simulink model "svlvspr1_schema_kyvadlo"  (R2018b)
settings: Solver=VariableStepAuto  StartTime=0.0  StopTime=10  RelTol=1e-3
values from neighbouring files (symbols this model uses):
  B = 1    [svlvspr1_skript_kyvadlo.m]
  g = 10    [svlvspr1_skript_kyvadlo.m]
  k1 = -2    [svlvspr1_skript_SVLVS.m]    (also in svlvspr1_skript_kyvadlo.m = 2)
  k2 = -4    [svlvspr1_skript_SVLVS.m]    (also in svlvspr1_skript_kyvadlo.m = 2.99)
  L = 10    [svlvspr1_skript_kyvadlo.m]
  m = 1    [svlvspr1_skript_kyvadlo.m]
  r = pi    (= 3.14159265359)    [svlvspr1_skript_SVLVS.m]    (also in svlvspr1_skript_kyvadlo.m = 1.0471975512)
settings Model: Creator=Evka  LastModifiedBy=Evka

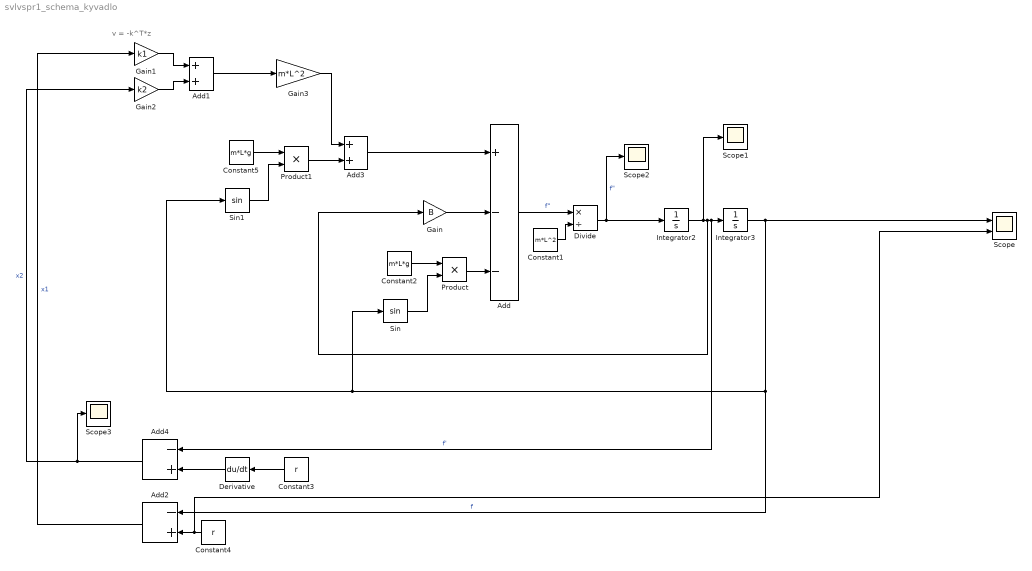
== system svlvspr1_schema_kyvadlo ==
  note: v = -k^T*z
  Add : Sum  Inputs=+--
  Add1 : Sum
  Add2 : Sum  Inputs=-+
  Add3 : Sum
  Add4 : Sum  Inputs=-+
  Constant1 : Constant  Value=m*L^2
  Constant2 : Constant  Value=m*L*g
  Constant3 : Constant  Value=r
  Constant4 : Constant  Value=r
  Constant5 : Constant  Value=m*L*g
  Derivative : Derivative
  Divide : Product  Inputs=*/
  Gain : Gain  Gain=B
  Gain1 : Gain  Gain=k1
  Gain2 : Gain  Gain=k2
  Gain3 : Gain  Gain=m*L^2
  Integrator2 : Integrator
  Integrator3 : Integrator
  Product : Product
  Product1 : Product
  Scope : Scope  NumInputPorts=2
  Scope1 : Scope
  Scope2 : Scope
  Scope3 : Scope
  Sin : Trigonometry
  Sin1 : Trigonometry
  wires:
  Add3/1 -> Add/1
  Divide/1 -> Scope2/1, Integrator2/1  "f\""
  Integrator2/1 -> Scope1/1, Gain/1, Add4/1, Integrator3/1  "f'"
  Integrator3/1 -> Add2/1, Sin1/1, Sin/1, Scope/1  "f"
  Gain/1 -> Add/2
  Add/1 -> Divide/1  "f\""
  Constant1/1 -> Divide/2
  Constant2/1 -> Product/1
  Product/1 -> Add/3
  Sin/1 -> Product/2
  Gain1/1 -> Add1/1
  Gain2/1 -> Add1/2
  Add1/1 -> Gain3/1
  Constant5/1 -> Product1/1
  Sin1/1 -> Product1/2
  Product1/1 -> Add3/2
  Gain3/1 -> Add3/1
  Constant4/1 -> Scope/2, Add2/2
  Add2/1 -> Gain1/1  "x1"
  Constant3/1 -> Derivative/1
  Add4/1 -> Scope3/1, Gain2/1  "x2"
  Derivative/1 -> Add4/2
